simulink model "Mechanical_model_01"  (R2017a)
settings: Solver=VariableStepAuto  StartTime=0.0  StopTime=10.0  RelTol=1e-3
settings Model: Creator=uidn7735  LastModifiedBy=uidn7735

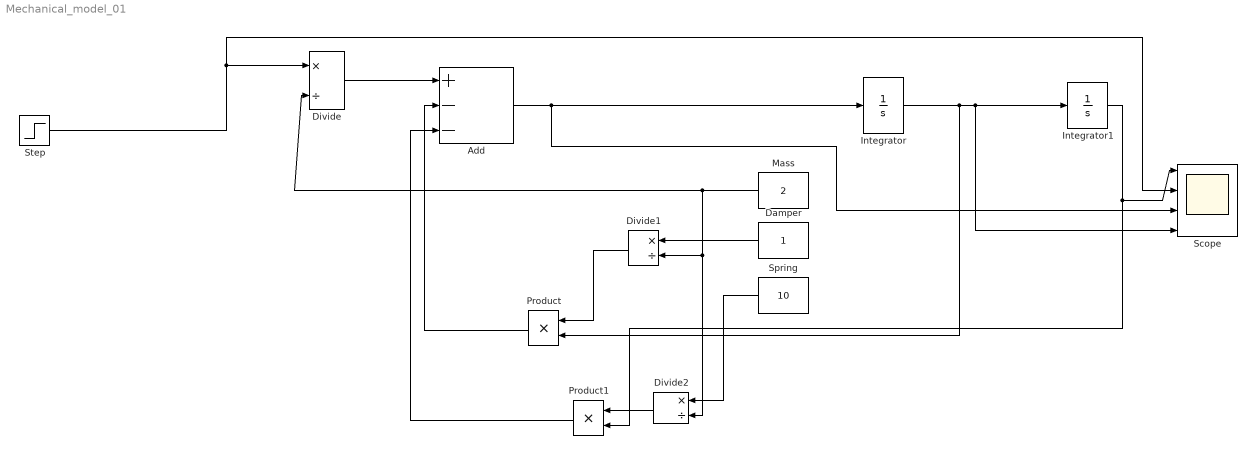
== system Mechanical_model_01 ==
  Add : Sum  Inputs=+--
  Damper : Constant
  Divide : Product  Inputs=*/
  Divide1 : Product  Inputs=*/
  Divide2 : Product  Inputs=*/
  Integrator : Integrator
  Integrator1 : Integrator
  Mass : Constant  Value=2
  Product : Product
  Product1 : Product
  Scope : Scope  NumInputPorts=4
  Spring : Constant  Value=10
  Step : Step  Before=1  After=0  SampleTime=0
  wires:
  Mass/1 -> Divide2/2, Divide1/2, Divide/2
  Step/1 -> Scope/2, Divide/1
  Divide/1 -> Add/1
  Add/1 -> Scope/3, Integrator/1
  Integrator/1 -> Product/2, Scope/4, Integrator1/1
  Damper/1 -> Divide1/1
  Divide1/1 -> Product/1
  Product/1 -> Add/2
  Spring/1 -> Divide2/1
  Divide2/1 -> Product1/1
  Integrator1/1 -> Scope/1, Product1/2
  Product1/1 -> Add/3
